simulink model "model_fully_coupled"  (R2021a)
settings: Solver=ode4  StartTime=0.0  StopTime=4  FixedStep=1e-2  RelTol=1e-3
values from neighbouring files (symbols this model uses):
  C_1 = [0.7887 -0.2113 -0.5774; -0.2113 0.7887 -0.5774; 0.5774 0.5774 0.5774]    [parameter.m]
  C_2 = [-0.2113 -0.5774 0.7887; 0.7887 -0.5774 -0.2113; 0.5774 0.5774 0.5774]    [parameter.m]
  C_3 = [-0.5774 0.7887 -0.2113; -0.5774 -0.2113 0.7887; 0.5774 0.5774 0.5774]    [parameter.m]
  d_1 = d    (= 4e-07)    [parameter.m]
  d_2 = d    (= 4e-07)    [parameter.m]
  d_3 = d    (= 4e-07)    [parameter.m]
  F = [0;0;0]    [parameter.m]
  g_s_1 = C_1(1:3,1)    [parameter.m]
  g_s_2 = C_2(1:3,1)    [parameter.m]
  g_s_3 = C_3(1:3,1)    [parameter.m]
  I = [1 0 0;0 1 0;0 0 1]    [parameter.m]
  I_hub_Bc = [550 0.1045 -0.0840; 0.1045 650 0.0001; -0.0840 0.0001 650]    [parameter.m]
  I_rw1_Wc1 = [1.5915E-4 0 1.54E-10; 0 0.8594E-4 0; 1.54E-10 0 0.8594E-4]    [parameter.m]
  I_rw1_Wc1_ = [0 -J_13_1 J_12_1; -J_13_1 (-2*J_23_1) (J_22_1-J_33_1); J_12_1 (J_22_1-J_33_1) (-2*J_23_1)]    [parameter.m]
  I_rw2_Wc2 = [1.5915E-4 0 1.54E-10; 0 0.8594E-4 0; 1.54E-10 0 0.8594E-4]    [parameter.m]
  I_rw2_Wc2_ = [0 -J_13_2 J_12_2; -J_13_2 (-2*J_23_2) (J_22_2-J_33_2); J_12_2 (J_22_2-J_33_2) (-2*J_23_2)]    [parameter.m]
  I_rw3_Wc3 = [1.5915E-4 0 1.54E-10; 0 0.8594E-4 0; 1.54E-10 0 0.8594E-4]    [parameter.m]
  I_rw3_Wc3_ = [0 -J_13_3 J_12_3; -J_13_3 (-2*J_23_3) (J_22_3-J_33_3); J_12_3 (J_22_3-J_33_3) (-2*J_23_3)]    [parameter.m]
  J_11_1 = I_rw1_Wc1(1,1)    [parameter.m]
  J_11_2 = I_rw2_Wc2(1,1)    [parameter.m]
  J_11_3 = I_rw3_Wc3(1,1)    [parameter.m]
  J_12_1 = I_rw1_Wc1(1,2)    [parameter.m]
  J_12_2 = I_rw2_Wc2(1,2)    [parameter.m]
  J_12_3 = I_rw3_Wc3(1,2)    [parameter.m]
  J_13_1 = I_rw1_Wc1(1,3)    [parameter.m]
  J_13_2 = I_rw2_Wc2(1,3)    [parameter.m]
  J_13_3 = I_rw3_Wc3(1,3)    [parameter.m]
  J_22_1 = I_rw1_Wc1(2,2)    [parameter.m]
  J_22_2 = I_rw2_Wc2(2,2)    [parameter.m]
  J_22_3 = I_rw3_Wc3(2,2)    [parameter.m]
  J_23_1 = I_rw1_Wc1(2,3)    [parameter.m]
  J_23_2 = I_rw2_Wc2(2,3)    [parameter.m]
  J_23_3 = I_rw3_Wc3(2,3)    [parameter.m]
  J_33_1 = I_rw1_Wc1(3,3)    [parameter.m]
  J_33_2 = I_rw2_Wc2(3,3)    [parameter.m]
  J_33_3 = I_rw3_Wc3(3,3)    [parameter.m]
  m_hub = 644    [parameter.m]
  m_rw_1 = m_rw(1)    [parameter.m]
  m_rw_2 = m_rw(2)    [parameter.m]
  m_rw_3 = m_rw(3)    [parameter.m]
  m_sc = 680    [parameter.m]
  OMEGA_1 = OMEGA(1)    [parameter.m]
  OMEGA_2 = OMEGA(2)    [parameter.m]
  OMEGA_3 = OMEGA(3)    [parameter.m]
  omega_BN = [omega ; omega; omega]    [parameter.m]
  r_Bc_B = [1e-2; -2e-2; 10e-2]    [parameter.m]
  r_BN = [0;0;0]    [parameter.m]
  r_W1_B = [0.6309; -0.1691; 0.4619]    [parameter.m]
  r_W2_B = [-0.1691; 0.6309; 0.4619]    [parameter.m]
  r_W3_B = [-0.4619; -0.4619; 0.4619]    [parameter.m]
  sigma_BN = [sigma; sigma; sigma]    [parameter.m]
  u_s_1 = u_s(1)    [parameter.m]
  u_s_2 = u_s(2)    [parameter.m]
  u_s_3 = u_s(3)    [parameter.m]
  w_2_1 = C_1(1:3,2)    [parameter.m]
  w_2_2 = C_2(1:3,2)    [parameter.m]
  w_2_3 = C_3(1:3,2)    [parameter.m]
  w_3_1 = C_1(1:3,3)    [parameter.m]
  w_3_2 = C_2(1:3,3)    [parameter.m]
  w_3_3 = C_3(1:3,3)    [parameter.m]
undefined symbols (not defined in the file or in its folder): deg, magnitude, rad, s
libraries: aerolibconvert2 x4, sharedutil x1, aerolibutil x1
(part 3 of 3)

== system model_fully_coupled/r_double_dot_BN/c_double_dot/r_dprime_Wci_B/r_Wci_B'/Subsystem2/r'_Wc3_B ==
  d_3 : Inport
  Product4 : Product
  1 : Outport
  wires:
  d_3/1 -> Product4/1
  Product4/1 -> 1/1
  [w_2_3_prime] -> Product4/2

== system model_fully_coupled/r_double_dot_BN/c_double_dot/r_dprime_Wci_B/r_Wci_B'/Subsystem2/r_Wc3_B ==
  r_W3_B : Inport
  d_3 : Inport  Port=2
  w_2_3 : Inport  Port=3
  Add2 : Sum
  Product2 : Product
  1 : Outport
  wires:
  Add2/1 -> 1/1
  d_3/1 -> Product2/1
  w_2_3/1 -> Product2/2
  Product2/1 -> Add2/2
  r_W3_B/1 -> Add2/1

== system model_fully_coupled/r_double_dot_BN/c_double_dot/r_dprime_Wci_B/r_Wci_B'/Subsystem/r"_Wc1_B/Subsystem1 ==
  1 : Inport
  Demux : Demux  Outputs=3
  skew : MATLAB Function  TreatAsAtomicUnit=on
  "skew " : Outport
  wires:
  1/1 -> Demux/1
  Demux/3 -> skew/3(a_3)
  Demux/2 -> skew/2(a_2)
  Demux/1 -> skew/1(a_1)
  skew/1(skew) -> "skew "/1

== system model_fully_coupled/r_double_dot_BN/c_double_dot/r_dprime_Wci_B/r_Wci_B'/Subsystem1/r"_Wc2_B/Subsystem1 ==
  1 : Inport
  Demux : Demux  Outputs=3
  skew : MATLAB Function  TreatAsAtomicUnit=on
  "skew " : Outport
  wires:
  1/1 -> Demux/1
  Demux/3 -> skew/3(a_3)
  Demux/2 -> skew/2(a_2)
  Demux/1 -> skew/1(a_1)
  skew/1(skew) -> "skew "/1

== system model_fully_coupled/r_double_dot_BN/c_double_dot/r_dprime_Wci_B/r_Wci_B'/Subsystem2/r"_Wc3_B/Subsystem1 ==
  1 : Inport
  Demux : Demux  Outputs=3
  skew : MATLAB Function  TreatAsAtomicUnit=on
  "skew " : Outport
  wires:
  1/1 -> Demux/1
  Demux/3 -> skew/3(a_3)
  Demux/2 -> skew/2(a_2)
  Demux/1 -> skew/1(a_1)
  skew/1(skew) -> "skew "/1

== matlab function model_fully_coupled/r_double_dot_BN/c_double_dot/r_dprime_Wci_B/r_Wci_B'/Subsystem1/Subsystem1/skew ==
  data: a_1 input; skew output; a_2 input; a_3 input
function skew = fcn(a_1, a_2, a_3)

skew = [0 -a_3 a_2; a_3 0 -a_1; -a_2 a_1 0];

== matlab function model_fully_coupled/r_double_dot_BN/c_double_dot/r_dprime_Wci_B/r_Wci_B'/Subsystem1/Subsystem2/skew ==
  data: a_1 input; skew output; a_2 input; a_3 input
function skew = fcn(a_1, a_2, a_3)

skew = [0 -a_3 a_2; a_3 0 -a_1; -a_2 a_1 0];

== matlab function model_fully_coupled/r_double_dot_BN/c_double_dot/r_dprime_Wci_B/r_Wci_B'/Subsystem2/Subsystem1/skew ==
  data: a_1 input; skew output; a_2 input; a_3 input
function skew = fcn(a_1, a_2, a_3)

skew = [0 -a_3 a_2; a_3 0 -a_1; -a_2 a_1 0];

== matlab function model_fully_coupled/r_double_dot_BN/c_double_dot/r_dprime_Wci_B/r_Wci_B'/Subsystem2/Subsystem2/skew ==
  data: a_1 input; skew output; a_2 input; a_3 input
function skew = fcn(a_1, a_2, a_3)

skew = [0 -a_3 a_2; a_3 0 -a_1; -a_2 a_1 0];

== matlab function model_fully_coupled/H_sc_B/1/Subsystem1/skew ==
  data: a_1 input; skew output; a_2 input; a_3 input
function skew = fcn(a_1, a_2, a_3)

skew = [0 -a_3 a_2; a_3 0 -a_1; -a_2 a_1 0];

== matlab function model_fully_coupled/OMEGA_dot_i/1/2/4/Subsystem1/skew ==
  data: a_1 input; skew output; a_2 input; a_3 input
function skew = fcn(a_1, a_2, a_3)

skew = [0 -a_3 a_2; a_3 0 -a_1; -a_2 a_1 0];

== matlab function model_fully_coupled/OMEGA_dot_i/2/2/4/Subsystem1/skew ==
  data: a_1 input; skew output; a_2 input; a_3 input
function skew = fcn(a_1, a_2, a_3)

skew = [0 -a_3 a_2; a_3 0 -a_1; -a_2 a_1 0];

== matlab function model_fully_coupled/OMEGA_dot_i/3/2/4/Subsystem1/skew ==
  data: a_1 input; skew output; a_2 input; a_3 input
function skew = fcn(a_1, a_2, a_3)

skew = [0 -a_3 a_2; a_3 0 -a_1; -a_2 a_1 0];

== matlab function model_fully_coupled/r_double_dot_BN/c_double_dot/2/Subsystem1/skew ==
  data: a_1 input; skew output; a_2 input; a_3 input
function skew = fcn(a_1, a_2, a_3)

skew = [0 -a_3 a_2; a_3 0 -a_1; -a_2 a_1 0];

== matlab function model_fully_coupled/r_double_dot_BN/c_double_dot/Subsystem1/skew ==
  data: a_1 input; skew output; a_2 input; a_3 input
function skew = fcn(a_1, a_2, a_3)

skew = [0 -a_3 a_2; a_3 0 -a_1; -a_2 a_1 0];

== matlab function model_fully_coupled/body frame to inertial frame/MATLAB Function ==
  data: B input; N output; sigma_BN input
function N = fcn(B, sigma_BN)

dcm_NB = ConvertAttitude(sigma_BN, 'mrp', 'dcm');
dcm_BN = dcm_NB.';

N = dcm_BN * B;

== matlab function model_fully_coupled/sigma_dot_BN/Subsystem/skew ==
  data: a_1 input; skew output; a_2 input; a_3 input
function skew = fcn(a_1, a_2, a_3)

skew = [0 -a_3 a_2; a_3 0 -a_1; -a_2 a_1 0];

== matlab function model_fully_coupled/r_double_dot_BN/c_double_dot/r_dprime_Wci_B/r_Wci_B'/Subsystem/r"_Wc1_B/Subsystem1/skew ==
  data: a_1 input; skew output; a_2 input; a_3 input
function skew = fcn(a_1, a_2, a_3)

skew = [0 -a_3 a_2; a_3 0 -a_1; -a_2 a_1 0];

== matlab function model_fully_coupled/omega_dot_BN/2 /Subsystem1/skew ==
  data: a_1 input; skew output; a_2 input; a_3 input
function skew = fcn(a_1, a_2, a_3)

skew = [0 -a_3 a_2; a_3 0 -a_1; -a_2 a_1 0];

== matlab function model_fully_coupled/r_double_dot_BN/c_double_dot/r_dprime_Wci_B/r_Wci_B'/Subsystem1/r"_Wc2_B/Subsystem1/skew ==
  data: a_1 input; skew output; a_2 input; a_3 input
function skew = fcn(a_1, a_2, a_3)

skew = [0 -a_3 a_2; a_3 0 -a_1; -a_2 a_1 0];

== matlab function model_fully_coupled/r_double_dot_BN/c_double_dot/r_dprime_Wci_B/r_Wci_B'/Subsystem2/r"_Wc3_B/Subsystem1/skew ==
  data: a_1 input; skew output; a_2 input; a_3 input
function skew = fcn(a_1, a_2, a_3)

skew = [0 -a_3 a_2; a_3 0 -a_1; -a_2 a_1 0];

== matlab function model_fully_coupled/r_double_dot_BN/c_double_dot/r_dprime_Wci_B/r_Wci_B'/Subsystem/Subsystem1/skew ==
  data: a_1 input; skew output; a_2 input; a_3 input
function skew = fcn(a_1, a_2, a_3)

skew = [0 -a_3 a_2; a_3 0 -a_1; -a_2 a_1 0];

== matlab function model_fully_coupled/r_double_dot_BN/c_double_dot/3/Subsystem1/skew ==
  data: a_1 input; skew output; a_2 input; a_3 input
function skew = fcn(a_1, a_2, a_3)

skew = [0 -a_3 a_2; a_3 0 -a_1; -a_2 a_1 0];

== matlab function model_fully_coupled/r_double_dot_BN/c_double_dot/r_dprime_Wci_B/r_Wci_B'/Subsystem/Subsystem2/skew ==
  data: a_1 input; skew output; a_2 input; a_3 input
function skew = fcn(a_1, a_2, a_3)

skew = [0 -a_3 a_2; a_3 0 -a_1; -a_2 a_1 0];
